simulink model "segway_planar_linmod_no_L"  (R2023a)
settings: Solver=VariableStepAuto  StartTime=0.0  StopTime=10.0  RelTol=1e-3
values from neighbouring files (symbols this model uses):
  Cinp = eye(2)    [segway_ini.m]    (also in segway_planar_ini.m = 1)
  Cout = eye(2)    [segway_ini.m]    (also in segway_planar_ini.m = 1)
  Cr2w = Cw2r^-1    [segway_ini.m]    (also in segway_planar_ini.m)
  Cw2r = [p.r/2     p.r/2;          p.r/p.b, -p.r/p.b]    [segway_ini.m]    (also in segway_planar_ini.m = [p.r])
  p = get_segway_params()    [segway_ini.m]    (also in segway_planar_ini.m)
libraries: cstblocks x1
settings Model: Creator=Michael Peter  LastModifiedBy=Michael Peter

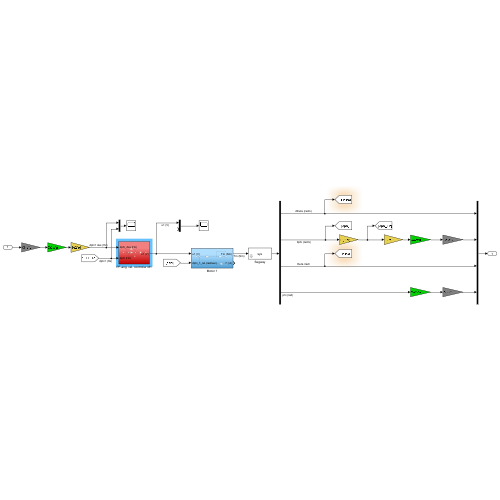
[thumbnail: Simulink's stored preview of the top-level diagram]
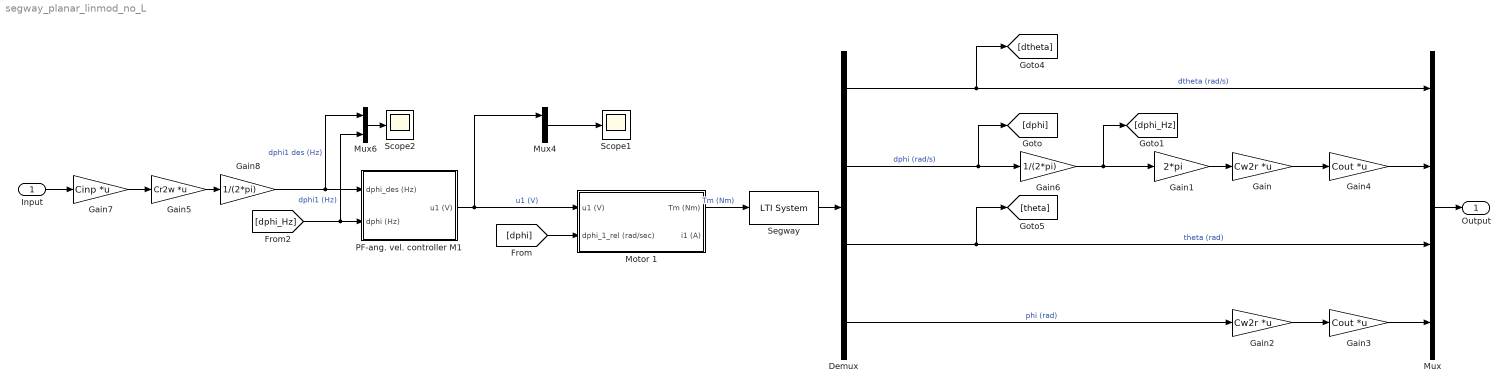
== system segway_planar_linmod_no_L ==
  Input : Inport
  Demux : Demux
  Gain : Gain  Gain=Cw2r  Multiplication=Matrix(K*u)
  Gain1 : Gain  Gain=2*pi
  Gain2 : Gain  Gain=Cw2r  Multiplication=Matrix(K*u)
  Gain3 : Gain  Gain=Cout  Multiplication=Matrix(K*u)
  Gain4 : Gain  Gain=Cout  Multiplication=Matrix(K*u)
  Gain5 : Gain  Gain=Cr2w  Multiplication=Matrix(K*u)
  Gain6 : Gain  Gain=1/(2*pi)
  Gain7 : Gain  Gain=Cinp  Multiplication=Matrix(K*u)
  Gain8 : Gain  Gain=1/(2*pi)
  Motor 1 : Subsystem
  Mux : Mux
  Mux4 : Mux  Inputs=2
  Mux6 : Mux  Inputs=2
  PF-ang. vel. controller M1 : Subsystem
  Scope1 : Scope
  Scope2 : Scope
  Segway : cstblocks/LTI System  sys=sys  IC=x0
  Output : Outport
  wires:
  Gain1/1 -> Gain/1
  Demux/2 -> Gain6/1, [dphi]  "dphi (rad/s)"
  Mux6/1 -> Scope2/1
  Gain3/1 -> Mux/4
  Demux/3 -> [theta], Mux/3  "theta (rad)"
  Gain4/1 -> Mux/2
  Gain7/1 -> Gain5/1
  Demux/1 -> [dtheta], Mux/1  "dtheta (rad/s)"
  Gain/1 -> Gain4/1
  Gain8/1 -> PF-ang. vel. controller M1/1(dphi_des (Hz)), Mux6/1  "dphi1 des (Hz)"
  PF-ang. vel. controller M1/1(u1 (V)) -> Motor 1/1(u1 (V)), Mux4/1  "u1 (V)"
  Motor 1/1(Tm (Nm)) -> Segway/1  "Tm (Nm)"
  Mux4/1 -> Scope1/1
  Input/1 -> Gain7/1
  Mux/1 -> Output/1
  Gain5/1 -> Gain8/1
  Segway/1 -> Demux/1
  [dphi] -> Motor 1/2(dphi_1_rel (rad/sec))
  Demux/4 -> Gain2/1  "phi (rad)"
  [dphi_Hz] -> PF-ang. vel. controller M1/2(dphi (Hz)), Mux6/2  "dphi1 (Hz)"
  Gain2/1 -> Gain3/1
  Gain6/1 -> Gain1/1, [dphi_Hz]

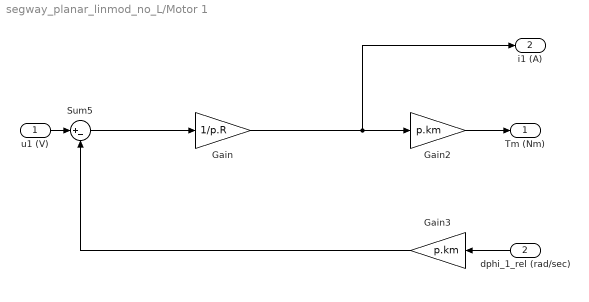
== system segway_planar_linmod_no_L/Motor 1 ==
  u1 (V) : Inport
  dphi_1_rel (rad/sec) : Inport  Port=2
  Gain : Gain  Gain=1/p.R
  Gain2 : Gain  Gain=p.km
  Gain3 : Gain  Gain=p.km
  Sum5 : Sum  Inputs=|+-
  Tm (Nm) : Outport
  i1 (A) : Outport  Port=2
  wires:
  Gain/1 -> i1 (A)/1, Gain2/1
  Gain3/1 -> Sum5/2
  u1 (V)/1 -> Sum5/1
  Sum5/1 -> Gain/1
  dphi_1_rel (rad/sec)/1 -> Gain3/1
  Gain2/1 -> Tm (Nm)/1

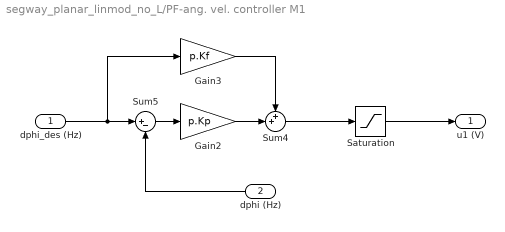
== system segway_planar_linmod_no_L/PF-ang. vel. controller M1 ==
  dphi_des (Hz) : Inport
  dphi (Hz) : Inport  Port=2
  Gain2 : Gain  Gain=p.Kp
  Gain3 : Gain  Gain=p.Kf
  Saturation : Saturate  UpperLimit=p.u_max  LowerLimit=p.u_min
  Sum4 : Sum  Inputs=++|
  Sum5 : Sum  Inputs=|+-
  u1 (V) : Outport
  wires:
  Sum5/1 -> Gain2/1
  dphi_des (Hz)/1 -> Gain3/1, Sum5/1
  dphi (Hz)/1 -> Sum5/2
  Gain3/1 -> Sum4/1
  Gain2/1 -> Sum4/2
  Sum4/1 -> Saturation/1
  Saturation/1 -> u1 (V)/1
